simulink model "simpleboat"  (R2022a)
settings: Solver=FixedStepAuto  StartTime=0.0  StopTime=10.0  FixedStep=0.01  RelTol=1e-3
libraries: etargetslib x1, slrealtimeiplib x1
settings Model: Creator=Pc  LastModifiedBy=Pc

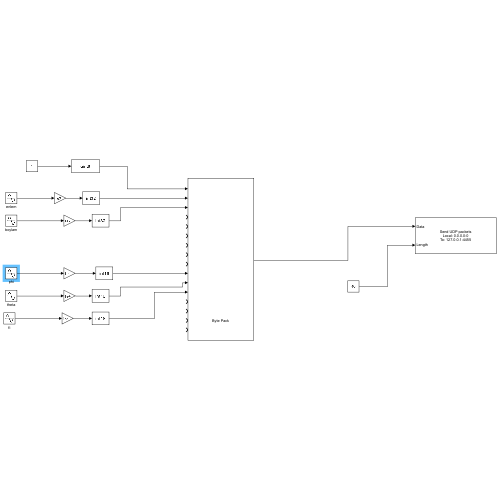
[thumbnail: Simulink's stored preview of the top-level diagram]
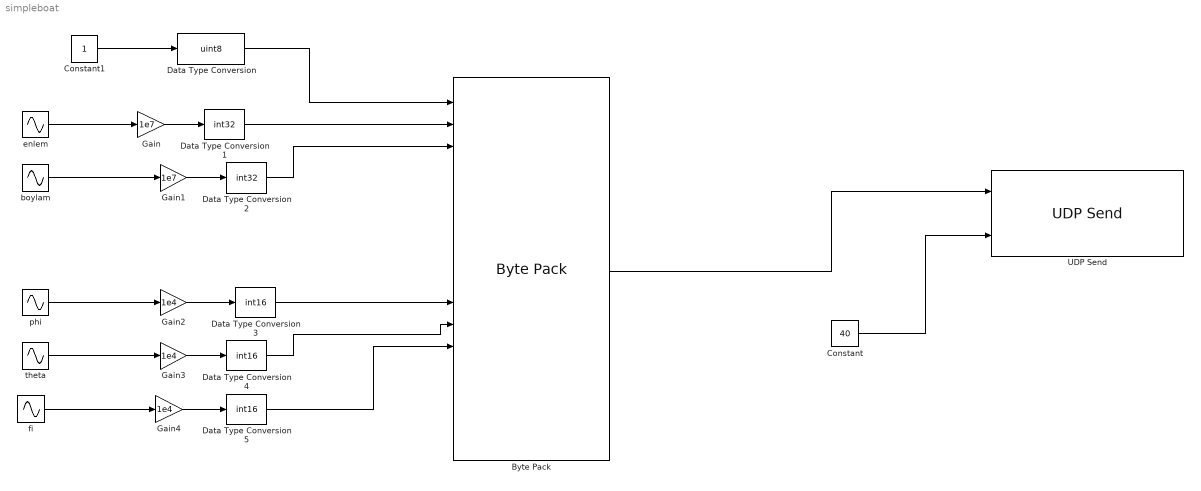
== system simpleboat ==
  Byte Pack : etargetslib/Byte Pack  datatypes=|  byteAlign=1
      | {'uint8'
      | ,'int32'
      | ,'int32'
      | ,'int16'
      | ,'int16'
      | ,'int16'
      | ,'int32'
      | ,'int32'
      | ,'int32'
      | ,'int16'
      | ,'int16'
      | ,'int16'
      | ,'int16'
      | ,'int16'
      | ,'int16'
      | ,'uint8'}
  Constant : Constant  Value=40
  Constant1 : Constant
  Data Type Conversion : DataTypeConversion  OutDataTypeStr=uint8  SaturateOnIntegerOverflow=off  RndMeth=Floor
  Data Type Conversion1 : DataTypeConversion  OutDataTypeStr=int32  SaturateOnIntegerOverflow=off  RndMeth=Floor
  Data Type Conversion2 : DataTypeConversion  OutDataTypeStr=int32  SaturateOnIntegerOverflow=off  RndMeth=Floor
  Data Type Conversion3 : DataTypeConversion  OutDataTypeStr=int16  SaturateOnIntegerOverflow=off  RndMeth=Floor
  Data Type Conversion4 : DataTypeConversion  OutDataTypeStr=int16  SaturateOnIntegerOverflow=off  RndMeth=Floor
  Data Type Conversion5 : DataTypeConversion  OutDataTypeStr=int16  SaturateOnIntegerOverflow=off  RndMeth=Floor
  Gain : Gain  Gain=1e7
  Gain1 : Gain  Gain=1e7
  Gain2 : Gain  Gain=1e4
  Gain3 : Gain  Gain=1e4
  Gain4 : Gain  Gain=1e4
  UDP Send : slrealtimeiplib/UDP Send  useHostTargetConn=off  toAddress='127.0.0.1'  toPort=4455  sampleTime=-1  enableMessage=off
      settings: SourceProductBaseCode=XP
  boylam : Sin  Amplitude=10000/111e3  Bias=42  Frequency=0.1  SampleTime=0
  enlem : Sin  Amplitude=10000/111e3  Bias=36  Frequency=0.1  SampleTime=0
  fi : Sin  Amplitude=0  Phase=pi/3  SampleTime=0
  phi : Sin  SampleTime=0
  theta : Sin  Amplitude=0  SampleTime=0
  wires:
  Byte Pack/1 -> UDP Send/1
  Constant/1 -> UDP Send/2
  Constant1/1 -> Data Type Conversion/1
  enlem/1 -> Gain/1
  boylam/1 -> Gain1/1
  Gain/1 -> Data Type Conversion1/1
  Gain1/1 -> Data Type Conversion2/1
  phi/1 -> Gain2/1
  theta/1 -> Gain3/1
  Gain3/1 -> Data Type Conversion4/1
  Gain2/1 -> Data Type Conversion3/1
  fi/1 -> Gain4/1
  Gain4/1 -> Data Type Conversion5/1
  Data Type Conversion/1 -> Byte Pack/1
  Data Type Conversion1/1 -> Byte Pack/2
  Data Type Conversion2/1 -> Byte Pack/3
  Data Type Conversion3/1 -> Byte Pack/10
  Data Type Conversion4/1 -> Byte Pack/11
  Data Type Conversion5/1 -> Byte Pack/12
